simulink model "ES106A_StHlthSigStc"  (R2013b)
settings: Solver=FixedStepDiscrete  SolverMode=SingleTasking  StartTime=0.0  StopTime=1  FixedStep=0.002  RelTol=1e-3
undefined symbols (not defined in the file): APPL10_CNT_U08, BITSPERBYTE_CNT_U08, ENOTOK_CNT_U08, EOK_CNT_U08, LOWRMASKVAL_CNT_U32, NROFCRCAREA_CNT_U08, NVMAVRGPOSN_CNT_U08, NvmGetErrSts1, NVMMAXPOSN_CNT_U08, NVMMINPOSN_CNT_U08, NVMSAMPLECNTRPOSN_CNT_U08, RAMMAXPOSN_CNT_U08, RAMMINPOSN_CNT_U08, RAMRAWPOSN_CNT_U08, SIGCNT_ULS_U08, SigStcPrmInst, STHLTHMAXVAL_CNT_U08, STHLTHOSAPPL_CNT_U16, StHlthTaskRef1, WORDSIZE_CNT_U08
libraries: simulink x43, NxtrNvM x4, NxtrMax x4, NxtrMin x4, FloatToFixd x3, NxtrLim x2
(part 3 of 5)

== system ES106A_StHlthSigStc/StHlthSigStc/ClrSigStcHlthData/ClrDataSample/Clear Nvm Data ==
  note: Clear all contents of NVM except the first byte. First byte shall remain untouched which keeps the CRC
  Action Port : ActionPort  ActionType=then
  Constant : Constant  Value=false  OutDataTypeStr=boolean
      settings: AttributesFormatString=%<OutDataTypeStr>
  Constant2 : Constant  Value=0*(1:225)  OutDataTypeStr=uint8
      settings: AttributesFormatString=%<OutDataTypeStr>
  CopyRight2 : Subsystem  Description=|  mask(Copyright Information){none=on}
      | Copyright info block.                                               
      |                                                                     
      | Place copyright information at the top of every subsystem in design.
      mask prompts: none "No parameters"
      mask help: Place copyright information at the top of every subsystem in design.
      mask Display:
      | NxtrConf = 'Nexteer Confidential';
      | 
      | sys = bdroot; %handle for the current model ("system")
      | first = get_param(sys,'Created');
      | first = first(end-3:end);  %year is last four digits
      | 
      | last = get_param(sys,'LastModifiedDate');
      | if isempty(last)
      |     last = datestr(now,'yyyy');
      | else
      |     last = last(end-3:end);
      | end
      | 
      | if strcmp(first,last)
      |     fprintf('%s -- Copyright %s Nexteer',NxtrConf,first)
      | else
      |     fprintf('%s -- %s%s- %s Nexteer',NxtrConf,char(169),first,last)
      | end
  Data Store Write1 : DataStoreWrite  DataStoreName=SigStcHistDataAry
  Data Store Write5 : DataStoreWrite  DataStoreName=VldNvm
  Set Ram Block Status : NxtrNvM/Set Ram Block Status  RequirementInfo={} %GIDa_3b942e49_0b20_480b_9dc6_15316d5aeb84  FuncName=Set Ram Block Status  NvMBlockName=SigStcHistDataAry  VoidFuncRtn=on  BlockChanged_DSN=NvMSRBS_BlockChanged  Return_DSN=NvMSRBS_Return1
      settings: AttributesFormatString=%<FuncName>
  WriteFlag : Constant  RequirementInfo={} %GIDa_b30764af_7e7b_4731_9fb4_92738979a70c  Value=true  OutDataTypeStr=boolean
      settings: AttributesFormatString=%<OutDataTypeStr>
  wires:
  Constant/1 -> Data Store Write5/1
  WriteFlag/1 -> Set Ram Block Status/1
  Constant2/1 -> Data Store Write1/1

== system ES106A_StHlthSigStc/StHlthSigStc/ClrSigStcHlthData/ClrDataSample/CopyRight2 ==

== system ES106A_StHlthSigStc/StHlthSigStc/ClrSigStcHlthData/ClrDataSample/Dont clear Nvm Data ==
  Action Port : ActionPort  ActionType=else
  CopyRight2 : Subsystem  Description=|  mask(Copyright Information){none=on}
      | Copyright info block.                                               
      |                                                                     
      | Place copyright information at the top of every subsystem in design.
      mask prompts: none "No parameters"
      mask help: Place copyright information at the top of every subsystem in design.
      mask Display:
      | NxtrConf = 'Nexteer Confidential';
      | 
      | sys = bdroot; %handle for the current model ("system")
      | first = get_param(sys,'Created');
      | first = first(end-3:end);  %year is last four digits
      | 
      | last = get_param(sys,'LastModifiedDate');
      | if isempty(last)
      |     last = datestr(now,'yyyy');
      | else
      |     last = last(end-3:end);
      | end
      | 
      | if strcmp(first,last)
      |     fprintf('%s -- Copyright %s Nexteer',NxtrConf,first)
      | else
      |     fprintf('%s -- %s%s- %s Nexteer',NxtrConf,char(169),first,last)
      | end

== system ES106A_StHlthSigStc/StHlthSigStc/ClrSigStcHlthData/ClrDataSample/For Iterator Subsystem ==
  "SigCnt " : Inport
  Add : Sum
  Assignment2 : Assignment  IndexMode=Zero-based  IndexOptions=Starting index (port)  Indices=1  OutputSizes=1
  Bus Selector2 : BusSelector  OutputSignals=RamStorgOffs
  Constant5 : Constant  Value=RAMMINPOSN_CNT_U08
  Constant6 : Constant  Value=STHLTHMAXVAL_CNT_U08  OutDataTypeStr=uint8
  CopyRight2 : Subsystem  Description=|  mask(Copyright Information){none=on}
      | Copyright info block.                                               
      |                                                                     
      | Place copyright information at the top of every subsystem in design.
      mask prompts: none "No parameters"
      mask help: Place copyright information at the top of every subsystem in design.
      mask Display:
      | NxtrConf = 'Nexteer Confidential';
      | 
      | sys = bdroot; %handle for the current model ("system")
      | first = get_param(sys,'Created');
      | first = first(end-3:end);  %year is last four digits
      | 
      | last = get_param(sys,'LastModifiedDate');
      | if isempty(last)
      |     last = datestr(now,'yyyy');
      | else
      |     last = last(end-3:end);
      | end
      | 
      | if strcmp(first,last)
      |     fprintf('%s -- Copyright %s Nexteer',NxtrConf,first)
      | else
      |     fprintf('%s -- %s%s- %s Nexteer',NxtrConf,char(169),first,last)
      | end
  Data Store Read3 : DataStoreRead  DataStoreName=SigStcPrmInst  DataStoreElements=SigStcPrmInst(:)
  Data Store Read4 : DataStoreRead  DataStoreName=RamBuf
  Data Store Write2 : DataStoreWrite  DataStoreName=RamBuf
  For Iterator : ForIterator  IterationSource=external  IndexMode=Zero-based
  Selector1 : Selector  IndexMode=Zero-based  InputPortWidth=22  IndexOptions=Index vector (port)  Indices=[1 3]  OutputSizes=1
  wires:
  "SigCnt "/1 -> For Iterator/1
  For Iterator/1 -> Selector1/2
  Selector1/1 -> Bus Selector2/1
  Data Store Read3/1 -> Selector1/1
  Bus Selector2/1 -> Add/1  "<RamStorgOffs>"
  Constant5/1 -> Add/2
  Add/1 -> Assignment2/3
  Data Store Read4/1 -> Assignment2/1
  Constant6/1 -> Assignment2/2
  Assignment2/1 -> Data Store Write2/1

== system ES106A_StHlthSigStc/StHlthSigStc/ClrSigStcHlthData/GetApplicationID/CopyRight2 ==

== system ES106A_StHlthSigStc/StHlthSigStc/GetSigStcHlthData/If Action Subsystem/CopyRight2 ==

== system ES106A_StHlthSigStc/StHlthSigStc/GetSigStcHlthData/If Action Subsystem1/CopyRight2 ==

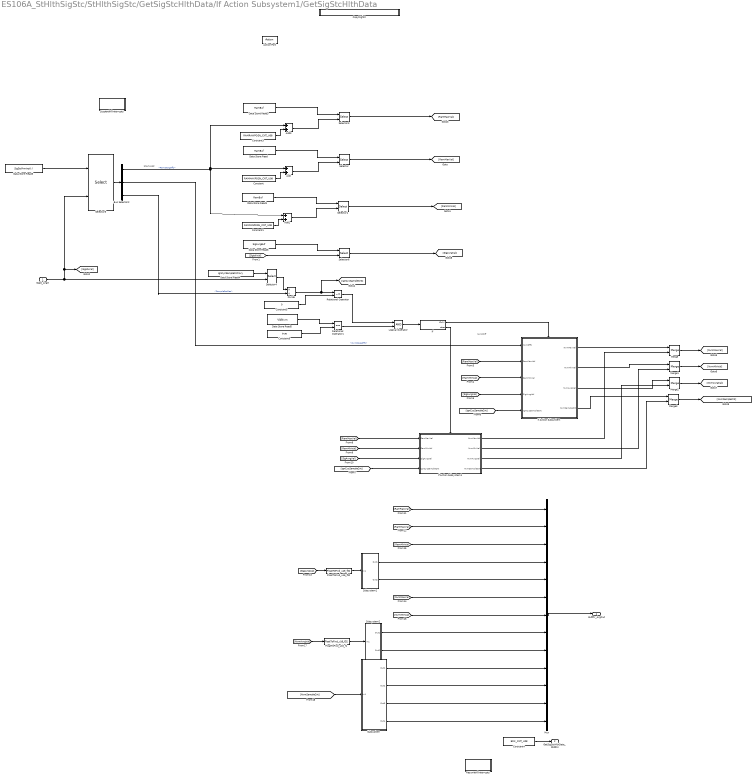
== system ES106A_StHlthSigStc/StHlthSigStc/GetSigStcHlthData/If Action Subsystem1/GetSigStcHlthData ==
  note: NVMOff
  note: StartAddr
  SigId_ArgIn : Inport
  Action Port : ActionPort  ActionType=then
  Add : Sum
  Add1 : Sum
  Add3 : Sum
  Bus Selector2 : BusSelector  OutputSignals=RamStorgOffs,NvmStorgOffs,SamplePerSec
  Constant : Constant  Value=RAMMAXPOSN_CNT_U08
  Constant1 : Constant  Value=RAMMINPOSN_CNT_U08
  Constant3 : Constant  Value=RAMRAWPOSN_CNT_U08
  Constant4 : Constant  Value=EOK_CNT_U08
  Constant5 : Constant  Value=0  OutDataTypeStr=uint32
      settings: AttributesFormatString=%<OutDataTypeStr>
  Constant6 : Constant  Value=true  OutDataTypeStr=boolean
      settings: AttributesFormatString=%<OutDataTypeStr>
  CopyRight2 : Subsystem  Description=|  mask(Copyright Information){none=on}
      | Copyright info block.                                               
      |                                                                     
      | Place copyright information at the top of every subsystem in design.
      mask prompts: none "No parameters"
      mask help: Place copyright information at the top of every subsystem in design.
      mask Display:
      | NxtrConf = 'Nexteer Confidential';
      | 
      | sys = bdroot; %handle for the current model ("system")
      | first = get_param(sys,'Created');
      | first = first(end-3:end);  %year is last four digits
      | 
      | last = get_param(sys,'LastModifiedDate');
      | if isempty(last)
      |     last = datestr(now,'yyyy');
      | else
      |     last = last(end-3:end);
      | end
      | 
      | if strcmp(first,last)
      |     fprintf('%s -- Copyright %s Nexteer',NxtrConf,first)
      | else
      |     fprintf('%s -- %s%s- %s Nexteer',NxtrConf,char(169),first,last)
      | end
  Data Store Read : DataStoreRead  DataStoreName=RamBuf
  Data Store Read1 : DataStoreRead  DataStoreName=RamBuf
  Data Store Read3 : DataStoreRead  DataStoreName=RamBuf
  Data Store Read4 : DataStoreRead  DataStoreName=IgnCycSampleCntrAry
  Data Store Read5 : DataStoreRead  DataStoreName=SigStcPrmInst  DataStoreElements=SigStcPrmInst(:)
  "Data Store Read5 " : DataStoreRead  DataStoreName=VldNvm
  Data Store Read6 : DataStoreRead  DataStoreName=SigAvrgBuf
  Divide : Product  Inputs=*/
  FloatToFixd_u16_f1 : FloatToFixd/FloatToFixd_u16_f32  Param1=9
  FloatToFixd_u16_f32 : FloatToFixd/FloatToFixd_u16_f32  Param1=9
  If : If  IfExpression=u1
  If Action Subsystem : Subsystem  TreatAsAtomicUnit=on
  If Action Subsystem1 : Subsystem  TreatAsAtomicUnit=on
  Logical Operator : Logic  AllPortsSameDT=off  OutDataTypeStr=boolean
  Merge{,1..3} (4 alike) : Merge
  Mux : Mux  Inputs=13
  Relational Operator : RelationalOperator  Operator=~=  OutDataTypeStr=boolean
  Relational Operator1 : RelationalOperator  Operator===  OutDataTypeStr=boolean
  ResumeAllInterrupts : Subsystem
  Selector : Selector  IndexMode=Zero-based  InputPortWidth=66  IndexOptions=Starting index (port)  Indices=[1 3]  OutputSizes=1
  Selector1 : Selector  IndexMode=Zero-based  InputPortWidth=66  IndexOptions=Starting index (port)  Indices=[1 3]  OutputSizes=1
  Selector3 : Selector  IndexMode=Zero-based  InputPortWidth=66  IndexOptions=Starting index (port)  Indices=[1 3]  OutputSizes=1
  Selector4 : Selector  IndexMode=Zero-based  InputPortWidth=22  IndexOptions=Starting index (port)  Indices=[1 3]  OutputSizes=1
  Selector5 : Selector  IndexMode=Zero-based  InputPortWidth=22  IndexOptions=Index vector (port)  Indices=[1 3]  OutputSizes=1
  Selector6 : Selector  IndexMode=Zero-based  InputPortWidth=22  IndexOptions=Starting index (port)  Indices=[1 3]  OutputSizes=1
  Subsystem : Subsystem
  Subsystem1 : Subsystem
  Subsystem2 : Subsystem
  SuspendAllInterrupts : Subsystem
  BufPtr_ArgOut : Outport
  GetSigStcHlthData_StdRtn : Outport  Port=2
  wires:
  Data Store Read/1 -> Selector/1
  Constant/1 -> Add/2
  Add/1 -> Selector/2
  Selector/1 -> [RamMaxVal]
  Data Store Read1/1 -> Selector1/1
  Constant1/1 -> Add1/2
  Add1/1 -> Selector1/2
  Selector1/1 -> [RamMinVal]
  Data Store Read3/1 -> Selector3/1
  Constant3/1 -> Add3/2
  Add3/1 -> Selector3/2
  Selector3/1 -> [RamRawVal]
  Bus Selector2/1 -> Add3/1, Add/1, Add1/1  "<RamStorgOffs>"
  SigId_ArgIn/1 -> [SigIdxVal], Selector5/2, Selector4/2
  Selector4/1 -> Divide/1
  Logical Operator/1 -> If/1
  If/1 -> If Action Subsystem/Action
  If/2 -> If Action Subsystem1/Action
  [RamMaxVal] -> If Action Subsystem/2(RamMaxVal)
  [RamMinVal] -> If Action Subsystem/3(RamMinVal)
  [IgnCycSampleCnt] -> If Action Subsystem/5(IgnCycSampleCnt)
  [IgnCycSampleCnt] -> If Action Subsystem1/4(IgnCycSampleCnt)
  [RamMinVal] -> If Action Subsystem1/2(RamMinVal)
  [RamMaxVal] -> If Action Subsystem1/1(RamMaxVal)
  If Action Subsystem/1(NvmMaxVal) -> Merge/1
  If Action Subsystem1/1(NvmMaxVal) -> Merge/2
  If Action Subsystem/2(NvmMinVal) -> Merge1/1
  If Action Subsystem/3(NvmAvrgVal) -> Merge2/1
  If Action Subsystem/4(NvmSampleCnt) -> Merge3/1
  If Action Subsystem1/2(NvmMinVal) -> Merge1/2
  If Action Subsystem1/4(NvmSampleCnt) -> Merge3/2
  Merge/1 -> [NvmMaxVal]
  Merge1/1 -> [NvmMinVal]
  Merge2/1 -> [NvmAvrgVal]
  Merge3/1 -> [NvmSampleCnt]
  [RamRawVal] -> Mux/1
  [RamMaxVal] -> Mux/2
  [RamMinVal] -> Mux/3
  [NvmMaxVal] -> Mux/6
  [NvmMinVal] -> Mux/7
  Subsystem/1(Out1) -> Mux/10
  Subsystem/2(Out2) -> Mux/11
  Subsystem/3(Out3) -> Mux/12
  Subsystem/4(Out4) -> Mux/13
  Mux/1 -> BufPtr_ArgOut/1
  [NvmSampleCnt] -> Subsystem/1(In1)
  Data Store Read5/1 -> Selector5/1
  Selector5/1 -> Bus Selector2/1
  Bus Selector2/2 -> If Action Subsystem/1(NvmOffs)  "<NvmStorgOffs>"
  Bus Selector2/3 -> Divide/2  "<SamplePerSec>"
  Divide/1 -> [IgnCycSampleCnt], Relational Operator/1
  Data Store Read4/1 -> Selector4/1
  Constant4/1 -> GetSigStcHlthData_StdRtn/1
  Constant5/1 -> Relational Operator/2
  Relational Operator/1 -> Logical Operator/1
  "Data Store Read5 "/1 -> Relational Operator1/1
  Relational Operator1/1 -> Logical Operator/2
  Constant6/1 -> Relational Operator1/2
  Data Store Read6/1 -> Selector6/1
  Selector6/1 -> [SigAvrgVal]
  Subsystem1/1(Out1) -> Mux/4
  [SigAvrgVal] -> If Action Subsystem1/3(SigAvrgVal)
  [SigAvrgVal] -> If Action Subsystem/4(SigAvrgVal)
  Subsystem2/1(Out1) -> Mux/8
  [SigIdxVal] -> Selector6/2
  If Action Subsystem1/3(NvmAvrgVal) -> Merge2/2
  [SigAvrgVal] -> FloatToFixd_u16_f32/1
  FloatToFixd_u16_f32/1 -> Subsystem1/1(In1)
  Subsystem1/2(Out2) -> Mux/5
  [NvmAvrgVal] -> FloatToFixd_u16_f1/1
  FloatToFixd_u16_f1/1 -> Subsystem2/1(In1)
  Subsystem2/2(Out2) -> Mux/9

== system ES106A_StHlthSigStc/StHlthSigStc/GetSigStcHlthData/If Action Subsystem1/If Action Subsystem ==
  Action Port : ActionPort  ActionType=else
  Constant : Constant  Value=ENOTOK_CNT_U08
  CopyRight2 : Subsystem  Description=|  mask(Copyright Information){none=on}
      | Copyright info block.                                               
      |                                                                     
      | Place copyright information at the top of every subsystem in design.
      mask prompts: none "No parameters"
      mask help: Place copyright information at the top of every subsystem in design.
      mask Display:
      | NxtrConf = 'Nexteer Confidential';
      | 
      | sys = bdroot; %handle for the current model ("system")
      | first = get_param(sys,'Created');
      | first = first(end-3:end);  %year is last four digits
      | 
      | last = get_param(sys,'LastModifiedDate');
      | if isempty(last)
      |     last = datestr(now,'yyyy');
      | else
      |     last = last(end-3:end);
      | end
      | 
      | if strcmp(first,last)
      |     fprintf('%s -- Copyright %s Nexteer',NxtrConf,first)
      | else
      |     fprintf('%s -- %s%s- %s Nexteer',NxtrConf,char(169),first,last)
      | end
  GetSigStcHlthData_StdRtn1 : Outport
  wires:
  Constant/1 -> GetSigStcHlthData_StdRtn1/1

== system ES106A_StHlthSigStc/StHlthSigStc/StHlthSigStcInit1/Check Applicability/Do Nothing ==
  note: /************************Do Nothing*******************************/
  Action Port : ActionPort  ActionType=else
  Subsystem5 : Subsystem  Description=|  mask(Copyright Information){none=on}
      | Copyright info block.                                               
      |                                                                     
      | Place copyright information at the top of every subsystem in design.
      mask prompts: none "No parameters"
      mask help: Place copyright information at the top of every subsystem in design.
      mask Display:
      | NxtrConf = 'Nexteer Confidential';
      | 
      | sys = bdroot; %handle for the current model ("system")
      | first = get_param(sys,'Created');
      | first = first(end-3:end);  %year is last four digits
      | 
      | last = get_param(sys,'LastModifiedDate');
      | if isempty(last)
      |     last = datestr(now,'yyyy');
      | else
      |     last = last(end-3:end);
      | end
      | 
      | if strcmp(first,last)
      |     fprintf('%s -- Copyright %s Nexteer',NxtrConf,first)
      | else
      |     fprintf('%s -- %s%s- %s Nexteer',NxtrConf,char(169),first,last)
      | end

== system ES106A_StHlthSigStc/StHlthSigStc/StHlthSigStcInit1/Check Applicability/Set Nvm Invalid ==
  Action Port : ActionPort  ActionType=then
  Constant : Constant  Value=false  OutDataTypeStr=boolean
      settings: AttributesFormatString=%<OutDataTypeStr>
  Data Store Write : DataStoreWrite  DataStoreName=VldNvm
  Subsystem5 : Subsystem  Description=|  mask(Copyright Information){none=on}
      | Copyright info block.                                               
      |                                                                     
      | Place copyright information at the top of every subsystem in design.
      mask prompts: none "No parameters"
      mask help: Place copyright information at the top of every subsystem in design.
      mask Display:
      | NxtrConf = 'Nexteer Confidential';
      | 
      | sys = bdroot; %handle for the current model ("system")
      | first = get_param(sys,'Created');
      | first = first(end-3:end);  %year is last four digits
      | 
      | last = get_param(sys,'LastModifiedDate');
      | if isempty(last)
      |     last = datestr(now,'yyyy');
      | else
      |     last = last(end-3:end);
      | end
      | 
      | if strcmp(first,last)
      |     fprintf('%s -- Copyright %s Nexteer',NxtrConf,first)
      | else
      |     fprintf('%s -- %s%s- %s Nexteer',NxtrConf,char(169),first,last)
      | end
  wires:
  Constant/1 -> Data Store Write/1

== system ES106A_StHlthSigStc/StHlthSigStc/StHlthSigStcInit1/Check Applicability/Subsystem5 ==

== system ES106A_StHlthSigStc/StHlthSigStc/StHlthSigStcInit1/Crc_CalculateCRC8/Copyright1 ==

== system ES106A_StHlthSigStc/StHlthSigStc/StHlthSigStcInit1/For Simulation Purpose/CopyRight2 ==

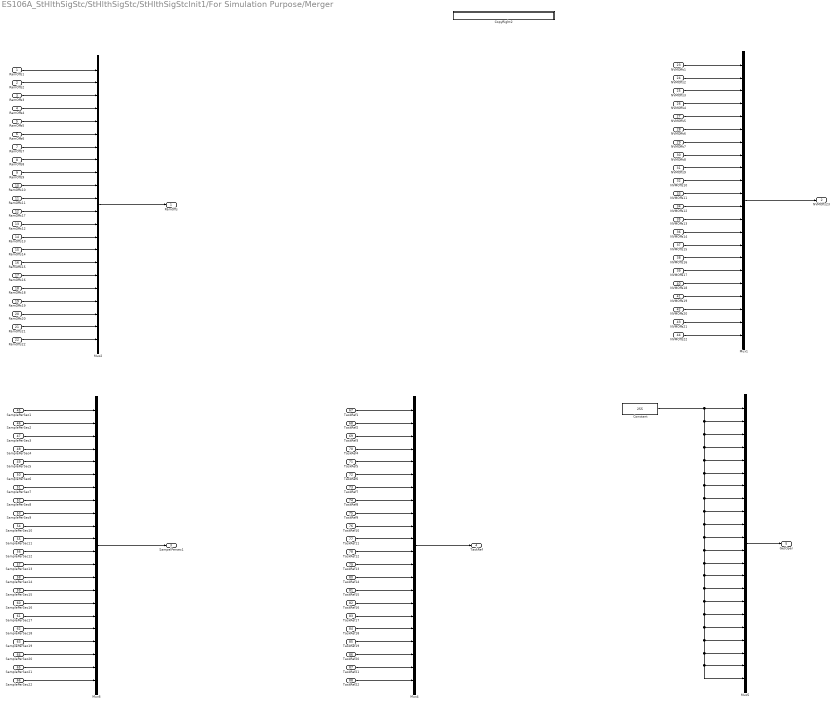
== system ES106A_StHlthSigStc/StHlthSigStc/StHlthSigStcInit1/For Simulation Purpose/Merger ==
  RamOffs1 : Inport
  RamOffs2 : Inport  Port=2
  RamOffs3 : Inport  Port=3
  RamOffs4 : Inport  Port=4
  RamOffs5 : Inport  Port=5
  RamOffs6 : Inport  Port=6
  RamOffs7 : Inport  Port=7
  RamOffs8 : Inport  Port=8
  RamOffs9 : Inport  Port=9
  RamOffs10 : Inport  Port=10
  RamOffs11 : Inport  Port=11
  RamOffs17 : Inport  Port=12
  RamOffs12 : Inport  Port=13
  RamOffs13 : Inport  Port=14
  RamOffs14 : Inport  Port=15
  RamOffs15 : Inport  Port=16
  RamOffs16 : Inport  Port=17
  RamOffs18 : Inport  Port=18
  RamOffs19 : Inport  Port=19
  RamOffs20 : Inport  Port=20
  RamOffs21 : Inport  Port=21
  RamOffs22 : Inport  Port=22
  NVMOffs1 : Inport  Port=23
  NVMOffs2 : Inport  Port=24
  NVMOffs3 : Inport  Port=25
  NVMOffs4 : Inport  Port=26
  NVMOffs5 : Inport  Port=27
  NVMOffs6 : Inport  Port=28
  NVMOffs7 : Inport  Port=29
  NVMOffs8 : Inport  Port=30
  NVMOffs9 : Inport  Port=31
  NVMOffs10 : Inport  Port=32
  NVMOffs11 : Inport  Port=33
  NVMOffs12 : Inport  Port=34
  NVMOffs13 : Inport  Port=35
  NVMOffs14 : Inport  Port=36
  NVMOffs15 : Inport  Port=37
  NVMOffs16 : Inport  Port=38
  NVMOffs17 : Inport  Port=39
  NVMOffs18 : Inport  Port=40
  NVMOffs19 : Inport  Port=41
  NVMOffs20 : Inport  Port=42
  NVMOffs21 : Inport  Port=43
  NVMOffs22 : Inport  Port=44
  SamplePerSec1 : Inport  Port=45
  SamplePerSec2 : Inport  Port=46
  SamplePerSec3 : Inport  Port=47
  SamplePerSec4 : Inport  Port=48
  SamplePerSec5 : Inport  Port=49
  SamplePerSec6 : Inport  Port=50
  SamplePerSec7 : Inport  Port=51
  SamplePerSec8 : Inport  Port=52
  SamplePerSec9 : Inport  Port=53
  SamplePerSec10 : Inport  Port=54
  SamplePerSec11 : Inport  Port=55
  SamplePerSec12 : Inport  Port=56
  SamplePerSec13 : Inport  Port=57
  SamplePerSec14 : Inport  Port=58
  SamplePerSec15 : Inport  Port=59
  SamplePerSec16 : Inport  Port=60
  SamplePerSec17 : Inport  Port=61
  SamplePerSec18 : Inport  Port=62
  SamplePerSec19 : Inport  Port=63
  SamplePerSec20 : Inport  Port=64
  SamplePerSec21 : Inport  Port=65
  SamplePerSec22 : Inport  Port=66
  TaskRef1 : Inport  Port=67
  TaskRef2 : Inport  Port=68
  TaskRef3 : Inport  Port=69
  TaskRef4 : Inport  Port=70
  TaskRef5 : Inport  Port=71
  TaskRef6 : Inport  Port=72
  TaskRef7 : Inport  Port=73
  TaskRef8 : Inport  Port=74
  TaskRef9 : Inport  Port=75
  TaskRef10 : Inport  Port=76
  TaskRef11 : Inport  Port=77
  TaskRef12 : Inport  Port=78
  TaskRef13 : Inport  Port=79
  TaskRef14 : Inport  Port=80
  TaskRef15 : Inport  Port=81
  TaskRef16 : Inport  Port=82
  TaskRef17 : Inport  Port=83
  TaskRef18 : Inport  Port=84
  TaskRef19 : Inport  Port=85
  TaskRef20 : Inport  Port=86
  TaskRef21 : Inport  Port=87
  TaskRef22 : Inport  Port=88
  Constant : Constant  Value=255  OutDataTypeStr=uint8
  CopyRight2 : Subsystem  Description=|  mask(Copyright Information){none=on}
      | Copyright info block.                                               
      |                                                                     
      | Place copyright information at the top of every subsystem in design.
      mask prompts: none "No parameters"
      mask help: Place copyright information at the top of every subsystem in design.
      mask Display:
      | NxtrConf = 'Nexteer Confidential';
      | 
      | sys = bdroot; %handle for the current model ("system")
      | first = get_param(sys,'Created');
      | first = first(end-3:end);  %year is last four digits
      | 
      | last = get_param(sys,'LastModifiedDate');
      | if isempty(last)
      |     last = datestr(now,'yyyy');
      | else
      |     last = last(end-3:end);
      | end
      | 
      | if strcmp(first,last)
      |     fprintf('%s -- Copyright %s Nexteer',NxtrConf,first)
      | else
      |     fprintf('%s -- %s%s- %s Nexteer',NxtrConf,char(169),first,last)
      | end
  Mux{1..2,4..6} (5 alike) : Mux  Inputs=22
  RamOffs : Outport
  NVMOffs23 : Outport  Port=2
  SampelPersec1 : Outport  Port=3
  TaskRef : Outport  Port=4
  GetOper : Outport  Port=5
  wires:
  RamOffs1/1 -> Mux2/1
  RamOffs2/1 -> Mux2/2
  Mux2/1 -> RamOffs/1
  RamOffs20/1 -> Mux2/20
  RamOffs19/1 -> Mux2/19
  RamOffs14/1 -> Mux2/15
  RamOffs15/1 -> Mux2/16
  RamOffs16/1 -> Mux2/17
  RamOffs18/1 -> Mux2/18
  RamOffs13/1 -> Mux2/14
  RamOffs12/1 -> Mux2/13
  NVMOffs1/1 -> Mux1/1
  NVMOffs2/1 -> Mux1/2
  Mux1/1 -> NVMOffs23/1
  NVMOffs5/1 -> Mux1/5
  NVMOffs14/1 -> Mux1/14
  NVMOffs4/1 -> Mux1/4
  NVMOffs6/1 -> Mux1/6
  NVMOffs15/1 -> Mux1/15
  NVMOffs7/1 -> Mux1/7
  NVMOffs16/1 -> Mux1/16
  NVMOffs8/1 -> Mux1/8
  NVMOffs13/1 -> Mux1/13
  NVMOffs17/1 -> Mux1/17
  NVMOffs9/1 -> Mux1/9
  NVMOffs3/1 -> Mux1/3
  NVMOffs18/1 -> Mux1/18
  NVMOffs10/1 -> Mux1/10
  NVMOffs19/1 -> Mux1/19
  NVMOffs11/1 -> Mux1/11
  NVMOffs20/1 -> Mux1/20
  NVMOffs12/1 -> Mux1/12
  Mux6/1 -> SampelPersec1/1
  SamplePerSec1/1 -> Mux6/1
  SamplePerSec2/1 -> Mux6/2
  SamplePerSec4/1 -> Mux6/4
  SamplePerSec5/1 -> Mux6/5
  SamplePerSec6/1 -> Mux6/6
  SamplePerSec3/1 -> Mux6/3
  SamplePerSec7/1 -> Mux6/7
  SamplePerSec8/1 -> Mux6/8
  SamplePerSec11/1 -> Mux6/11
  SamplePerSec9/1 -> Mux6/9
  SamplePerSec12/1 -> Mux6/12
  SamplePerSec10/1 -> Mux6/10
  SamplePerSec13/1 -> Mux6/13
  SamplePerSec14/1 -> Mux6/14
  SamplePerSec15/1 -> Mux6/15
  SamplePerSec16/1 -> Mux6/16
  SamplePerSec17/1 -> Mux6/17
  SamplePerSec18/1 -> Mux6/18
  SamplePerSec19/1 -> Mux6/19
  SamplePerSec20/1 -> Mux6/20
  Mux4/1 -> TaskRef/1
  TaskRef2/1 -> Mux4/2
  TaskRef1/1 -> Mux4/1
  TaskRef15/1 -> Mux4/15
  TaskRef16/1 -> Mux4/16
  TaskRef14/1 -> Mux4/14
  TaskRef4/1 -> Mux4/4
  TaskRef3/1 -> Mux4/3
  TaskRef17/1 -> Mux4/17
  TaskRef18/1 -> Mux4/18
  TaskRef13/1 -> Mux4/13
  TaskRef19/1 -> Mux4/19
  TaskRef6/1 -> Mux4/6
  TaskRef5/1 -> Mux4/5
  TaskRef10/1 -> Mux4/10
  TaskRef9/1 -> Mux4/9
  TaskRef7/1 -> Mux4/7
  TaskRef12/1 -> Mux4/12
  TaskRef20/1 -> Mux4/20
  TaskRef8/1 -> Mux4/8
  TaskRef11/1 -> Mux4/11
  Mux5/1 -> GetOper/1
  RamOffs4/1 -> Mux2/4
  RamOffs3/1 -> Mux2/3
  RamOffs9/1 -> Mux2/9
  RamOffs8/1 -> Mux2/8
  RamOffs7/1 -> Mux2/7
  RamOffs6/1 -> Mux2/6
  RamOffs10/1 -> Mux2/10
  RamOffs5/1 -> Mux2/5
  RamOffs11/1 -> Mux2/11
  RamOffs17/1 -> Mux2/12
  Constant/1 -> Mux5/2, Mux5/3, Mux5/22, Mux5/21, Mux5/20, Mux5/19, Mux5/18, Mux5/17, Mux5/16, Mux5/15, Mux5/14, Mux5/13, Mux5/12, Mux5/11, Mux5/10, Mux5/9, Mux5/8, Mux5/7, Mux5/6, Mux5/5, Mux5/4, Mux5/1
  RamOffs21/1 -> Mux2/21
  RamOffs22/1 -> Mux2/22
  NVMOffs21/1 -> Mux1/21
  NVMOffs22/1 -> Mux1/22
  SamplePerSec21/1 -> Mux6/21
  SamplePerSec22/1 -> Mux6/22
  TaskRef21/1 -> Mux4/21
  TaskRef22/1 -> Mux4/22

== system ES106A_StHlthSigStc/StHlthSigStc/StHlthSigStcInit1/Initialize Nvm/Subsystem5 ==

== system ES106A_StHlthSigStc/StHlthSigStc/StHlthSigStcInit1/Initialize the Minimum value for all SOH signals/Subsystem5 ==

== system ES106A_StHlthSigStc/StHlthSigStc/StHlthSigStcInit1/NvmNotVal/CopyRight2 ==

== system ES106A_StHlthSigStc/StHlthSigStc/StHlthSigStcInit1/Prepare a buffer for CRC calculation/CopyRight2 ==

== system ES106A_StHlthSigStc/StHlthSigStc/StHlthSigStcInit1/Prepare a buffer for CRC calculation/Iterator ==
  CrcData : Inport
  CrcOutrLoopCnt : Inport  Port=2
  Iterator : Inport  Port=3
  Add : Sum
  Assignment : Assignment  IndexMode=Zero-based  IndexOptions=Starting index (port)  Indices=1  OutputSizes=1
  Bitwise Operator : simulink/Logic and Bit Operations/Bitwise Operator  logicop=AND  UseBitMask=on  BitMask=bin2dec('11111111')  BitMaskRealWorld=Stored Integer
  CopyRight2 : Subsystem  Description=|  mask(Copyright Information){none=on}
      | Copyright info block.                                               
      |                                                                     
      | Place copyright information at the top of every subsystem in design.
      mask prompts: none "No parameters"
      mask help: Place copyright information at the top of every subsystem in design.
      mask Display:
      | NxtrConf = 'Nexteer Confidential';
      | 
      | sys = bdroot; %handle for the current model ("system")
      | first = get_param(sys,'Created');
      | first = first(end-3:end);  %year is last four digits
      | 
      | last = get_param(sys,'LastModifiedDate');
      | if isempty(last)
      |     last = datestr(now,'yyyy');
      | else
      |     last = last(end-3:end);
      | end
      | 
      | if strcmp(first,last)
      |     fprintf('%s -- Copyright %s Nexteer',NxtrConf,first)
      | else
      |     fprintf('%s -- %s%s- %s Nexteer',NxtrConf,char(169),first,last)
      | end
  Data Store Read : DataStoreRead  DataStoreName=CrcBuf
  Data Store Write : DataStoreWrite  DataStoreName=CrcBuf
  Data Type Conversion : DataTypeConversion  OutDataTypeStr=uint8
  Divide : Product  Inputs=**  OutDataTypeStr=Inherit: Inherit via back propagation
  Divide1 : Product  Inputs=**
  FirstCall = False1 : Constant  Value=BITSPERBYTE_CNT_U08
  FirstCall = False3 : Constant  Value=WORDSIZE_CNT_U08
  For Iterator : ForIterator  IterationSource=external  IterationLimit=WORDSIZE_CNT_U08  IndexMode=Zero-based
  Shift Arithmetic : ArithShift  BitShiftNumberSource=Input port  BitShiftNumber=8  BitShiftDirection=Right
      settings: InputPortMap=u0,p1
  wires:
  CrcData/1 -> Shift Arithmetic/1
  For Iterator/1 -> Add/2, Divide1/2
  CrcOutrLoopCnt/1 -> Divide/1
  Divide/1 -> Add/1
  FirstCall = False3/1 -> Divide/2
  Divide1/1 -> Shift Arithmetic/2
  Shift Arithmetic/1 -> Bitwise Operator/1
  Bitwise Operator/1 -> Data Type Conversion/1
  FirstCall = False1/1 -> Divide1/1
  Data Store Read/1 -> Assignment/1
  Assignment/1 -> Data Store Write/1
  Iterator/1 -> For Iterator/1
  Data Type Conversion/1 -> Assignment/2
  Add/1 -> Assignment/3

== system ES106A_StHlthSigStc/StHlthSigStc/StHlthStcPwrDwn/For Iterator Subsystem/CopyRight2 ==

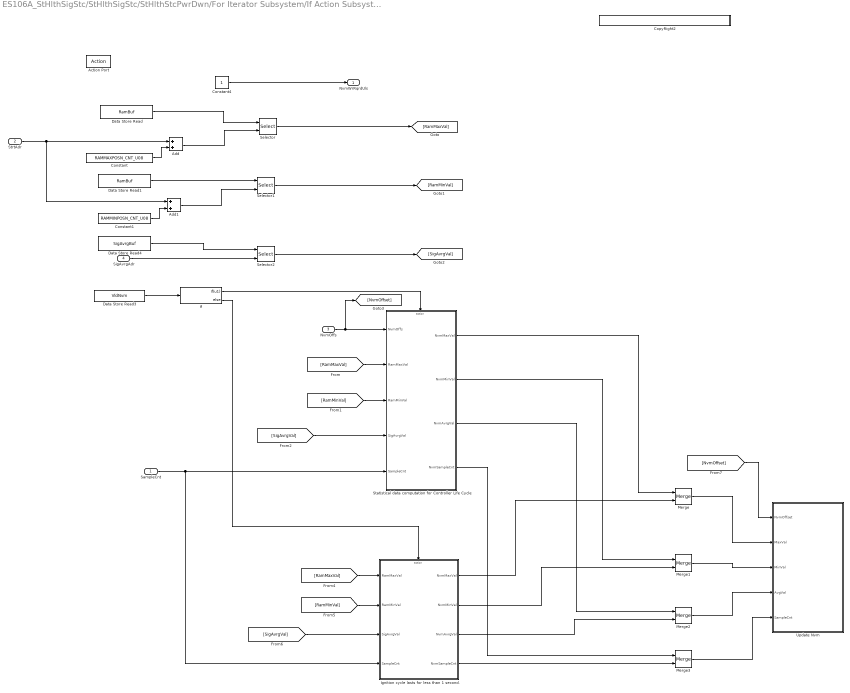
== system ES106A_StHlthSigStc/StHlthSigStc/StHlthStcPwrDwn/For Iterator Subsystem/If Action Subsystem ==
  SampleCnt : Inport
  StrtAdr : Inport  Port=2
  NvmOffs : Inport  Port=3
  SigAvrgAdr : Inport  Port=4
  Action Port : ActionPort  ActionType=then
  " Ignition cycle lasts for less than 1 second." : Subsystem  RequirementInfo={'linktype_rmi_doors' '0001022b (/ESG Group/FDD Module Requirements/EA4 Specific/ES106A_StHlthSigStc )' '#ES106A_45' 'true' 'REQ:ES106A_45' '' } %GIDa_88022069_4cda_42ee_afcb_4e354d20985b  TreatAsAtomicUnit=on
  Add : Sum
  Add1 : Sum
  Constant : Constant  Value=RAMMAXPOSN_CNT_U08  OutDataTypeStr=uint8
  Constant1 : Constant  Value=RAMMINPOSN_CNT_U08  OutDataTypeStr=uint8
  Constant4 : Constant
  CopyRight2 : Subsystem  Description=|  mask(Copyright Information){none=on}
      | Copyright info block.                                               
      |                                                                     
      | Place copyright information at the top of every subsystem in design.
      mask prompts: none "No parameters"
      mask help: Place copyright information at the top of every subsystem in design.
      mask Display:
      | NxtrConf = 'Nexteer Confidential';
      | 
      | sys = bdroot; %handle for the current model ("system")
      | first = get_param(sys,'Created');
      | first = first(end-3:end);  %year is last four digits
      | 
      | last = get_param(sys,'LastModifiedDate');
      | if isempty(last)
      |     last = datestr(now,'yyyy');
      | else
      |     last = last(end-3:end);
      | end
      | 
      | if strcmp(first,last)
      |     fprintf('%s -- Copyright %s Nexteer',NxtrConf,first)
      | else
      |     fprintf('%s -- %s%s- %s Nexteer',NxtrConf,char(169),first,last)
      | end
  Data Store Read : DataStoreRead  DataStoreName=RamBuf
  Data Store Read1 : DataStoreRead  DataStoreName=RamBuf
  Data Store Read3 : DataStoreRead  DataStoreName=VldNvm
  Data Store Read4 : DataStoreRead  DataStoreName=SigAvrgBuf
  If : If  IfExpression=u1
  Merge{,1..3} (4 alike) : Merge
  Selector : Selector  IndexMode=Zero-based  InputPortWidth=66  IndexOptions=Starting index (port)  Indices=[1 3]  OutputSizes=1
  Selector1 : Selector  IndexMode=Zero-based  InputPortWidth=66  IndexOptions=Starting index (port)  Indices=[1 3]  OutputSizes=1
  Selector2 : Selector  IndexMode=Zero-based  InputPortWidth=22  IndexOptions=Starting index (port)  Indices=[1 3]  OutputSizes=1
  Statistical data computation for Controller Life Cycle : Subsystem  RequirementInfo={'linktype_rmi_doors' '0001022b (/ESG Group/FDD Module Requirements/EA4 Specific/ES106A_StHlthSigStc )' '#ES106A_26' 'true' 'REQ:ES106A_26' '' ; 'linktype_rmi_doors' '0001022b (/ESG Group/FDD Module Requirements/EA4 Specific/ES106A_StHlthSigStc )' '#ES106A_28' 'true' 'REQ:ES106A_28' '' ; 'linktype_rmi_doors' '0001022b (/ESG Group/FDD Module Requirements/EA4 Specific/ES106A_StHlthSigStc )' '#ES106A_30' 'true' 'REQ:ES106A_30' '' ; 'linktype_rmi_doors' '0001022b (/ESG Group/FDD Module Requirements/EA4 Specific/ES106A_StHlthSigStc )' '#ES106A_31' 'true' 'REQ:ES106A_31' '' ; 'linktype_rmi_doors' '0001022b (/ESG Group/FDD Module Requirements/EA4 Specific/ES106A_StHlthSigStc )' '#ES106A_32' 'true' 'REQ:ES106A_32' '' ; 'linktype_rmi_doors' '0001022b (/ESG Group/FDD Module Requirements/EA4 Specific/ES106A_StHlthSigStc )' '#ES106A_33' 'true' 'REQ:ES106A_33' '' } %GIDa_8fc253a2_07f0_4162_a103_573a48d366c2  TreatAsAtomicUnit=on
  Update Nvm : Subsystem  RequirementInfo={'linktype_rmi_doors' '0001022b (/ESG Group/FDD Module Requirements/EA4 Specific/ES106A_StHlthSigStc )' '#ES106A_24' 'true' 'REQ:ES106A_24' '' ; 'linktype_rmi_doors' '0001022b (/ESG Group/FDD Module Requirements/EA4 Specific/ES106A_StHlthSigStc )' '#ES106A_42' 'true' 'REQ:ES106A_42' '' } %GIDa_8cf0ea3e_d97b_417e_afa9_a4336f2578f6
  NvmWrRqrdUls : Outport
  wires:
  Data Store Read/1 -> Selector/1
  Constant/1 -> Add/2
  Add/1 -> Selector/2
  Selector/1 -> [RamMaxVal]
  Data Store Read1/1 -> Selector1/1
  Constant1/1 -> Add1/2
  Add1/1 -> Selector1/2
  Selector1/1 -> [RamMinVal]
  Data Store Read4/1 -> Selector2/1
  StrtAdr/1 -> Add1/1, Add/1
  SigAvrgAdr/1 -> Selector2/2
  Selector2/1 -> [SigAvrgVal]
  Data Store Read3/1 -> If/1
  If/1 -> Statistical data computation for Controller Life Cycle/Action
  If/2 -> " Ignition cycle lasts for less than 1 second."/Action
  NvmOffs/1 -> [NvmOffset], Statistical data computation for Controller Life Cycle/1(NvmOffs)
  [RamMaxVal] -> " Ignition cycle lasts for less than 1 second."/1(RamMaxVal)
  [RamMinVal] -> " Ignition cycle lasts for less than 1 second."/2(RamMinVal)
  " Ignition cycle lasts for less than 1 second."/3(NvmAvrgVal) -> Merge2/2
  " Ignition cycle lasts for less than 1 second."/2(NvmMinVal) -> Merge1/2
  " Ignition cycle lasts for less than 1 second."/1(NvmMaxVal) -> Merge/2
  [RamMaxVal] -> Statistical data computation for Controller Life Cycle/2(RamMaxVal)
  [RamMinVal] -> Statistical data computation for Controller Life Cycle/3(RamMinVal)
  Statistical data computation for Controller Life Cycle/1(NvmMaxVal) -> Merge/1
  Statistical data computation for Controller Life Cycle/2(NvmMinVal) -> Merge1/1
  Statistical data computation for Controller Life Cycle/3(NvmAvrgVal) -> Merge2/1
  SampleCnt/1 -> " Ignition cycle lasts for less than 1 second."/4(SampleCnt), Statistical data computation for Controller Life Cycle/5(SampleCnt)
  " Ignition cycle lasts for less than 1 second."/4(NvmSampleCnt) -> Merge3/2
  Statistical data computation for Controller Life Cycle/4(NvmSampleCnt) -> Merge3/1
  Constant4/1 -> NvmWrRqrdUls/1
  Merge/1 -> Update Nvm/2(MaxVal)
  Merge1/1 -> Update Nvm/3(MinVal)
  Merge2/1 -> Update Nvm/4(AvgVal)
  Merge3/1 -> Update Nvm/5(SampleCnt)
  [NvmOffset] -> Update Nvm/1(NvmOffset)
  [SigAvrgVal] -> " Ignition cycle lasts for less than 1 second."/3(SigAvrgVal)
  [SigAvrgVal] -> Statistical data computation for Controller Life Cycle/4(SigAvrgVal)

== system ES106A_StHlthSigStc/StHlthSigStc/StHlthStcPwrDwn/If Action Subsystem1/CopyRight2 ==

== system ES106A_StHlthSigStc/StHlthSigStc/UpdStHlthStcData/Call Non Trusted Function /CopyRight2 ==

== system ES106A_StHlthSigStc/StHlthSigStc/UpdStHlthStcData/Call Non Trusted Function /For Iterator Subsystem ==
  note: TaskId which depends on OS layer is used to figure out
      | which tasks run and compare against TaskId_ArgIn
  note: Offset is used to update the RAMbuffer Index
  note: Function pointer will be used in code to get Signal Helath Status.
      | For simulation purpose,signal health status is directly given
      | as input instead of function pointer.
  TaskId_ArgIn : Inport
  SigCnt : Inport  Port=2
  StHlthSig : Inport  Port=3
  Bus Selector2 : BusSelector  OutputSignals=GetStHlthDataOper,TaskRef,RamStorgOffs
  CopyRight2 : Subsystem  Description=|  mask(Copyright Information){none=on}
      | Copyright info block.                                               
      |                                                                     
      | Place copyright information at the top of every subsystem in design.
      mask prompts: none "No parameters"
      mask help: Place copyright information at the top of every subsystem in design.
      mask Display:
      | NxtrConf = 'Nexteer Confidential';
      | 
      | sys = bdroot; %handle for the current model ("system")
      | first = get_param(sys,'Created');
      | first = first(end-3:end);  %year is last four digits
      | 
      | last = get_param(sys,'LastModifiedDate');
      | if isempty(last)
      |     last = datestr(now,'yyyy');
      | else
      |     last = last(end-3:end);
      | end
      | 
      | if strcmp(first,last)
      |     fprintf('%s -- Copyright %s Nexteer',NxtrConf,first)
      | else
      |     fprintf('%s -- %s%s- %s Nexteer',NxtrConf,char(169),first,last)
      | end
  Data Store Read2 : DataStoreRead  DataStoreName=SigStcPrmInst  DataStoreElements=SigStcPrmInst(:)
  Data Type Conversion : DataTypeConversion  OutDataTypeStr=uint8
  For Iterator : ForIterator  IterationSource=external  IterationLimit=2  IndexMode=Zero-based
  If Action Subsystem2 : Subsystem  TreatAsAtomicUnit=on
  If Task Id matches : If  NumInputs=2  IfExpression=u1 == u2
  Selector1 : Selector  IndexMode=Zero-based  InputPortWidth=22  IndexOptions=Index vector (port)  Indices=[1 3]  OutputSizes=1
  Subsystem2 : Subsystem
  wires:
  Selector1/1 -> Bus Selector2/1
  For Iterator/1 -> Subsystem2/3(SigIdx), Selector1/2
  TaskId_ArgIn/1 -> If Task Id matches/2
  Bus Selector2/1 -> Subsystem2/1(FunPtr)  "<GetStHlthDataOper>"
  Bus Selector2/2 -> Data Type Conversion/1  "<TaskRef>"
  Bus Selector2/3 -> Subsystem2/2(RAMOffset)  "<RamStorgOffs>"
  If Task Id matches/2 -> If Action Subsystem2/Action
  Data Store Read2/1 -> Selector1/1
  SigCnt/1 -> For Iterator/1
  Data Type Conversion/1 -> If Task Id matches/1
  If Task Id matches/1 -> Subsystem2/Action
  StHlthSig/1 -> Subsystem2/4(StHlthSig)

== system ES106A_StHlthSigStc/StHlthSigStc/UpdStHlthStcData/GetApplicationID/CopyRight2 ==

== system ES106A_StHlthSigStc/StHlthSigStc/UpdStHlthStcData/UpdDataSample/CopyRight2 ==

== system ES106A_StHlthSigStc/StHlthSigStc/UpdStHlthStcData/UpdDataSample/For Iterator Subsystem ==
  note: TaskId which depends on OS layer is used to figure out
      | which tasks run and compare against TaskId_ArgIn
  note: Offset is used to update the RAMbuffer Index
  note: Function pointer will be used in code to get Signal Helath Status.
      | For simulation purpose,signal health status is directly given
      | as input instead of function pointer.
  TaskId_ArgIn : Inport
  SigCnt : Inport  Port=2
  StHlthSig : Inport  Port=3
  Bus Selector2 : BusSelector  OutputSignals=GetStHlthDataOper,TaskRef,RamStorgOffs
  CopyRight2 : Subsystem  Description=|  mask(Copyright Information){none=on}
      | Copyright info block.                                               
      |                                                                     
      | Place copyright information at the top of every subsystem in design.
      mask prompts: none "No parameters"
      mask help: Place copyright information at the top of every subsystem in design.
      mask Display:
      | NxtrConf = 'Nexteer Confidential';
      | 
      | sys = bdroot; %handle for the current model ("system")
      | first = get_param(sys,'Created');
      | first = first(end-3:end);  %year is last four digits
      | 
      | last = get_param(sys,'LastModifiedDate');
      | if isempty(last)
      |     last = datestr(now,'yyyy');
      | else
      |     last = last(end-3:end);
      | end
      | 
      | if strcmp(first,last)
      |     fprintf('%s -- Copyright %s Nexteer',NxtrConf,first)
      | else
      |     fprintf('%s -- %s%s- %s Nexteer',NxtrConf,char(169),first,last)
      | end
  Data Store Read2 : DataStoreRead  DataStoreName=SigStcPrmInst  DataStoreElements=SigStcPrmInst(:)
  Data Type Conversion : DataTypeConversion  OutDataTypeStr=uint8
  For Iterator : ForIterator  IterationSource=external  IterationLimit=2  IndexMode=Zero-based
  If Action Subsystem2 : Subsystem  TreatAsAtomicUnit=on
  If Task Id matches : If  NumInputs=2  IfExpression=u1 == u2
  Selector1 : Selector  IndexMode=Zero-based  InputPortWidth=22  IndexOptions=Index vector (port)  Indices=[1 3]  OutputSizes=1
  Subsystem2 : Subsystem
  wires:
  Selector1/1 -> Bus Selector2/1
  For Iterator/1 -> Subsystem2/3(SigIdx), Selector1/2
  TaskId_ArgIn/1 -> If Task Id matches/2
  Bus Selector2/1 -> Subsystem2/1(FunPtr)  "<GetStHlthDataOper>"
  Bus Selector2/2 -> Data Type Conversion/1  "<TaskRef>"
  Bus Selector2/3 -> Subsystem2/2(RAMOffset)  "<RamStorgOffs>"
  If Task Id matches/2 -> If Action Subsystem2/Action
  Data Store Read2/1 -> Selector1/1
  SigCnt/1 -> For Iterator/1
  Data Type Conversion/1 -> If Task Id matches/1
  If Task Id matches/1 -> Subsystem2/Action
  StHlthSig/1 -> Subsystem2/4(StHlthSig)

== system ES106A_StHlthSigStc/StHlthSigStc/ClrSigStcHlthData/Call Non Trusted Function/Clear Nvm Data/CopyRight2 ==

== system ES106A_StHlthSigStc/StHlthSigStc/ClrSigStcHlthData/Call Non Trusted Function/Dont clear Nvm Data/CopyRight2 ==

== system ES106A_StHlthSigStc/StHlthSigStc/ClrSigStcHlthData/Call Non Trusted Function/For Iterator Subsystem/CopyRight2 ==

== system ES106A_StHlthSigStc/StHlthSigStc/ClrSigStcHlthData/ClrDataSample/Clear Nvm Data/CopyRight2 ==

== system ES106A_StHlthSigStc/StHlthSigStc/ClrSigStcHlthData/ClrDataSample/Dont clear Nvm Data/CopyRight2 ==

== system ES106A_StHlthSigStc/StHlthSigStc/ClrSigStcHlthData/ClrDataSample/For Iterator Subsystem/CopyRight2 ==

== system ES106A_StHlthSigStc/StHlthSigStc/GetSigStcHlthData/If Action Subsystem1/GetSigStcHlthData/CopyRight2 ==

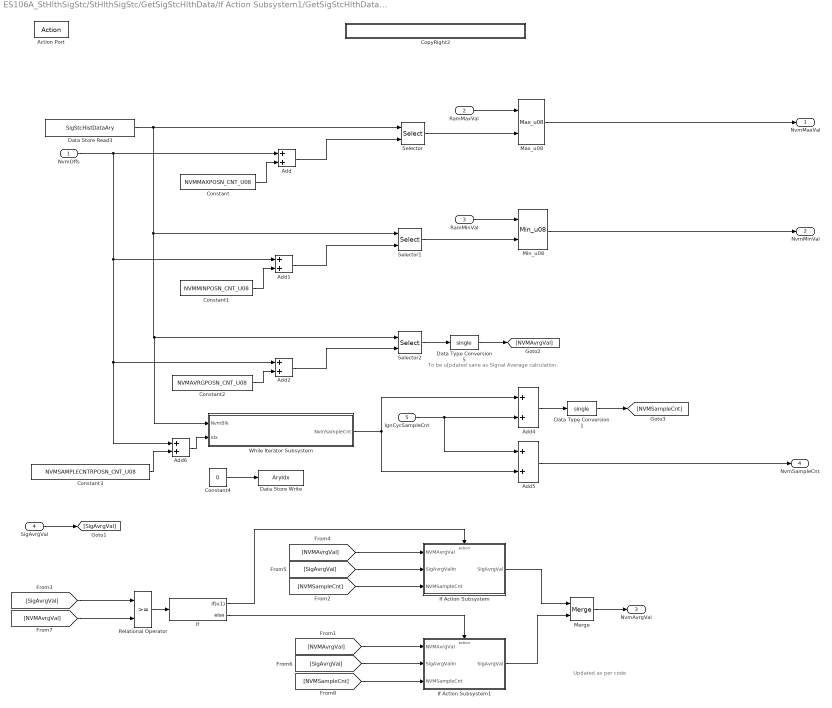
== system ES106A_StHlthSigStc/StHlthSigStc/GetSigStcHlthData/If Action Subsystem1/GetSigStcHlthData/If Action Subsystem ==
  note: To be u[pdated sane as Signal Average calculation.
  note: Updated as per code
  NvmOffs : Inport
  RamMaxVal : Inport  Port=2
  RamMinVal : Inport  Port=3
  SigAvrgVal : Inport  Port=4
  IgnCycSampleCnt : Inport  Port=5
  Action Port : ActionPort  ActionType=then
  Add{,1..2,4..6} (6 alike) : Sum
  Constant : Constant  Value=NVMMAXPOSN_CNT_U08
  Constant1 : Constant  Value=NVMMINPOSN_CNT_U08
  Constant2 : Constant  Value=NVMAVRGPOSN_CNT_U08
  Constant3 : Constant  Value=NVMSAMPLECNTRPOSN_CNT_U08
  Constant4 : Constant  Value=0
  CopyRight2 : Subsystem  Description=|  mask(Copyright Information){none=on}
      | Copyright info block.                                               
      |                                                                     
      | Place copyright information at the top of every subsystem in design.
      mask prompts: none "No parameters"
      mask help: Place copyright information at the top of every subsystem in design.
      mask Display:
      | NxtrConf = 'Nexteer Confidential';
      | 
      | sys = bdroot; %handle for the current model ("system")
      | first = get_param(sys,'Created');
      | first = first(end-3:end);  %year is last four digits
      | 
      | last = get_param(sys,'LastModifiedDate');
      | if isempty(last)
      |     last = datestr(now,'yyyy');
      | else
      |     last = last(end-3:end);
      | end
      | 
      | if strcmp(first,last)
      |     fprintf('%s -- Copyright %s Nexteer',NxtrConf,first)
      | else
      |     fprintf('%s -- %s%s- %s Nexteer',NxtrConf,char(169),first,last)
      | end
  Data Store Read3 : DataStoreRead  DataStoreName=SigStcHistDataAry
  Data Store Write : DataStoreWrite  DataStoreName=AryIdx
  Data Type Conversion1 : DataTypeConversion  OutDataTypeStr=single
  Data Type Conversion5 : DataTypeConversion  OutDataTypeStr=single
  If : If  IfExpression=u1
  If Action Subsystem : Subsystem  TreatAsAtomicUnit=on
  If Action Subsystem1 : Subsystem  TreatAsAtomicUnit=on
  Max_u08 : NxtrMax/Max_u08  SFunctionSpec="uint8 y1 = Max_u08( uint8 u1,  uint8 u2)"
      settings: AttributesFormatString=%<Name>
  Merge : Merge
  Min_u08 : NxtrMin/Min_u08  SFunctionSpec="uint8 y1 = Min_u08( uint8 u1,  uint8 u2)"  ShowSpec=off
      settings: AttributesFormatString=%<Name>
  Relational Operator : RelationalOperator  OutDataTypeStr=boolean
  Selector : Selector  IndexMode=Zero-based  InputPortWidth=225  IndexOptions=Starting index (port)  Indices=[1 3]  OutputSizes=1
  Selector1 : Selector  IndexMode=Zero-based  InputPortWidth=225  IndexOptions=Starting index (port)  Indices=[1 3]  OutputSizes=1
  Selector2 : Selector  IndexMode=Zero-based  InputPortWidth=225  IndexOptions=Starting index (port)  Indices=[1 3]  OutputSizes=1
  While Iterator Subsystem : Subsystem  TreatAsAtomicUnit=on
  NvmMaxVal : Outport
  NvmMinVal : Outport  Port=2
  NvmAvrgVal : Outport  Port=3
  NvmSampleCnt : Outport  Port=4
  wires:
  Constant/1 -> Add/2
  Add/1 -> Selector/2
  Constant1/1 -> Add1/2
  Add1/1 -> Selector1/2
  NvmOffs/1 -> Add6/1, Add2/1, Add1/1, Add/1
  Constant2/1 -> Add2/2
  Add2/1 -> Selector2/2
  RamMaxVal/1 -> Max_u08/1
  Selector/1 -> Max_u08/2
  Max_u08/1 -> NvmMaxVal/1
  RamMinVal/1 -> Min_u08/1
  Selector1/1 -> Min_u08/2
  Min_u08/1 -> NvmMinVal/1
  Selector2/1 -> Data Type Conversion5/1
  IgnCycSampleCnt/1 -> Add5/1, Add4/2
  While Iterator Subsystem/1(NvmSampleCnt) -> Add4/1, Add5/2
  Add5/1 -> NvmSampleCnt/1
  Add4/1 -> Data Type Conversion1/1
  Constant3/1 -> Add6/2
  Add6/1 -> While Iterator Subsystem/2(Idx)
  Constant4/1 -> Data Store Write/1
  Data Store Read3/1 -> Selector2/1, While Iterator Subsystem/1(NvmBlk), Selector1/1, Selector/1
  Relational Operator/1 -> If/1
  If/1 -> If Action Subsystem/Action
  If/2 -> If Action Subsystem1/Action
  Merge/1 -> NvmAvrgVal/1
  If Action Subsystem/1(SigAvrgVal) -> Merge/1
  If Action Subsystem1/1(SigAvrgVal) -> Merge/2
  [NVMSampleCnt] -> If Action Subsystem/3(NVMSampleCnt)
  [SigAvrgVal] -> If Action Subsystem1/2(SigAvrgValIn)
  [SigAvrgVal] -> If Action Subsystem/2(SigAvrgValIn)
  [NVMAvrgVal] -> If Action Subsystem/1(NVMAvrgVal)
  [NVMAvrgVal] -> If Action Subsystem1/1(NVMAvrgVal)
  [SigAvrgVal] -> Relational Operator/1
  [NVMAvrgVal] -> Relational Operator/2
  [NVMSampleCnt] -> If Action Subsystem1/3(NVMSampleCnt)
  SigAvrgVal/1 -> [SigAvrgVal]
  Data Type Conversion5/1 -> [NVMAvrgVal]
  Data Type Conversion1/1 -> [NVMSampleCnt]

== system ES106A_StHlthSigStc/StHlthSigStc/GetSigStcHlthData/If Action Subsystem1/GetSigStcHlthData/If Action Subsystem1 ==
  RamMaxVal : Inport
  RamMinVal : Inport  Port=2
  SigAvrgVal : Inport  Port=3
  IgnCycSampleCnt : Inport  Port=4
  Action Port : ActionPort  ActionType=else
  CopyRight2 : Subsystem  Description=|  mask(Copyright Information){none=on}
      | Copyright info block.                                               
      |                                                                     
      | Place copyright information at the top of every subsystem in design.
      mask prompts: none "No parameters"
      mask help: Place copyright information at the top of every subsystem in design.
      mask Display:
      | NxtrConf = 'Nexteer Confidential';
      | 
      | sys = bdroot; %handle for the current model ("system")
      | first = get_param(sys,'Created');
      | first = first(end-3:end);  %year is last four digits
      | 
      | last = get_param(sys,'LastModifiedDate');
      | if isempty(last)
      |     last = datestr(now,'yyyy');
      | else
      |     last = last(end-3:end);
      | end
      | 
      | if strcmp(first,last)
      |     fprintf('%s -- Copyright %s Nexteer',NxtrConf,first)
      | else
      |     fprintf('%s -- %s%s- %s Nexteer',NxtrConf,char(169),first,last)
      | end
  NvmMaxVal : Outport
  NvmMinVal : Outport  Port=2
  NvmAvrgVal : Outport  Port=3
  NvmSampleCnt : Outport  Port=4
  wires:
  RamMaxVal/1 -> NvmMaxVal/1
  RamMinVal/1 -> NvmMinVal/1
  IgnCycSampleCnt/1 -> NvmSampleCnt/1
  SigAvrgVal/1 -> NvmAvrgVal/1

== system ES106A_StHlthSigStc/StHlthSigStc/GetSigStcHlthData/If Action Subsystem1/GetSigStcHlthData/ResumeAllInterrupts ==

== system ES106A_StHlthSigStc/StHlthSigStc/GetSigStcHlthData/If Action Subsystem1/GetSigStcHlthData/Subsystem ==
  In1 : Inport  OutDataTypeStr=uint32
  Bitwise Operator : simulink/Logic and Bit Operations/Bitwise Operator  logicop=AND  UseBitMask=on  BitMask=bin2dec('111111110000000000000000')  BitMaskRealWorld=Stored Integer
  Bitwise Operator1 : simulink/Logic and Bit Operations/Bitwise Operator  logicop=AND  UseBitMask=on  BitMask=bin2dec('1111111100000000')  BitMaskRealWorld=Stored Integer
  Bitwise Operator2 : simulink/Logic and Bit Operations/Bitwise Operator  logicop=AND  UseBitMask=on  BitMask=bin2dec('11111111')  BitMaskRealWorld=Stored Integer
  CopyRight2 : Subsystem  Description=|  mask(Copyright Information){none=on}
      | Copyright info block.                                               
      |                                                                     
      | Place copyright information at the top of every subsystem in design.
      mask prompts: none "No parameters"
      mask help: Place copyright information at the top of every subsystem in design.
      mask Display:
      | NxtrConf = 'Nexteer Confidential';
      | 
      | sys = bdroot; %handle for the current model ("system")
      | first = get_param(sys,'Created');
      | if(isempty(first))
      |     first = datestr(now,'yyyy');
      | else
      |     first = first(end-3:end);  %year is last four digits
      | end
      | 
      | last = get_param(sys,'LastModifiedDate');
      | if isempty(last)
      |     last = datestr(now,'yyyy');
      | else
      |     last = last(end-3:end);
      | end
      | 
      | if strcmp(first,last)
      |     fprintf('%s -- Copyright %s Nexteer',NxtrConf,first)
      | else
      |     fprintf('%s -- %s%s- %s Nexteer',NxtrConf,char(169),first,last)
      | end
  Data Type Conversion{,1..3} (4 alike) : DataTypeConversion  OutDataTypeStr=uint8
  Shift Arithmetic : ArithShift  BitShiftNumber=SHIFTFAC16_ULS_U08  BitShiftDirection=Right
  Shift Arithmetic1 : ArithShift  BitShiftNumber=SHIFTFAC24_ULS_U08  BitShiftDirection=Right
  Shift Arithmetic2 : ArithShift  BitShiftNumber=SHIFTFAC8_ULS_U08  BitShiftDirection=Right
  Out1 : Outport
  Out2 : Outport  Port=2
  Out3 : Outport  Port=3
  Out4 : Outport  Port=4
  wires:
  Shift Arithmetic2/1 -> Data Type Conversion2/1
  In1/1 -> Shift Arithmetic1/1, Bitwise Operator/1, Bitwise Operator2/1, Bitwise Operator1/1
  Bitwise Operator2/1 -> Data Type Conversion3/1
  Bitwise Operator/1 -> Shift Arithmetic/1
  Shift Arithmetic/1 -> Data Type Conversion1/1
  Shift Arithmetic1/1 -> Data Type Conversion/1
  Bitwise Operator1/1 -> Shift Arithmetic2/1
  Data Type Conversion/1 -> Out1/1
  Data Type Conversion1/1 -> Out2/1
  Data Type Conversion2/1 -> Out3/1
  Data Type Conversion3/1 -> Out4/1
